simulink model "c01_MainAdc"  (R2024a)
settings: Solver=FixedStepDiscrete  StartTime=0.0  StopTime=1  FixedStep=mSim.dTime  MaxStep=Define.sModelSampleTime  RelTol=7.1420e-05
undefined symbols (not defined in the file): C01ISENS, C01VSENS, C01VTEST
libraries: Lib_LPF x1
settings Model: Creator=user  LastModifiedBy=admin
settings SolverCC: MaxConsecutiveZCs=10000  ZeroCrossAlgorithm=Adaptive  AlgebraicLoopSolver=TrustRegion
settings DataIOCC: SaveOutput=off  DSMLogging=off  InspectSignalLogs=on  SaveTime=off  SignalLoggingName=logsout_Validator
settings OptimizationCC: BlockReduction=off  DefaultParameterBehavior=Inlined  UseDivisionForNetSlopeComputation=UseDivisionForReciprocalsOfIntegersOnly  GainParamInheritBuiltInType=on  UseFloatMulNetSlope=on  DefaultUnderspecifiedDataType=single  InlineInvariantSignals=on  BitwiseOrLogicalOp=Logical operator  PassReuseOutputArgsAs=Individual arguments  EfficientFloat2IntCast=on  LifeSpan=Inf  OptimizeBlockOrder=speed  DifferentSizesBufferReuse=on  EfficientTunableParamExpr=on
settings DebuggingCC: SignalInfNanChecking=error  SignalRangeChecking=error  ReadBeforeWriteMsg=EnableAllAsError  WriteAfterWriteMsg=EnableAllAsError  WriteAfterReadMsg=EnableAllAsError  AlgebraicLoopMsg=error  ArtificialAlgebraicLoopMsg=error  SaveWithDisabledLinksMsg=error  SaveWithParameterizedLinksMsg=error  BlockPriorityViolationMsg=error  SolverPrmCheckMsg=error  InheritedTsInSrcMsg=error  SingleTaskRateTransMsg=error  TasksWithSamePriorityMsg=error  SigSpecEnsureSampleTimeMsg=error  CheckMatrixSingularityMsg=error  IntegerOverflowMsg=error  ParameterUnderflowMsg=error  ParameterPrecisionLossMsg=error  ParameterTunabilityLossMsg=error  UnderSpecifiedDataTypeMsg=error  UnnecessaryDatatypeConvMsg=warning  VectorMatrixConversionMsg=error  SignalLabelMismatchMsg=error  UnconnectedInputMsg=error  UnconnectedOutputMsg=error  UnconnectedLineMsg=error  SFcnCompatibilityMsg=error  UniqueDataStoreMsg=error  BusObjectLabelMismatch=error  RootOutportRequireBusObject=error  AssertControl=DisableAll  ModelReferenceIOMismatchMessage=error  UnknownTsInhSupMsg=error  ModelReferenceDataLoggingMessage=error  ModelReferenceSymbolNameMessage=none  StateNameClashWarn=warning  StrictBusMsg=ErrorOnBusTreatedAsVector  NonBusSignalsTreatedAsBus=error  SFInvalidInputDataAccessInChartInitDiag=error  SFTransitionOutsideNaturalParentDiag=error  SFUnreachableExecutionPathDiag=error  SFUndirectedBroadcastEventsDiag=error  SFTransitionActionBeforeConditionDiag=error  SFTemporalDelaySmallerThanSampleTimeDiag=error  SFSelfTransitionDiag=error  SFExecutionAtInitializationDiag=error  IntegerSaturationMsg=error  UnitsInconsistencyMsg=none  VariantConditionMismatch=error
settings HardwareCC: ProdBitPerChar=16  ProdBitPerInt=16  ProdBitPerPointer=32  ProdBitPerSizeT=32  ProdBitPerPtrDiffT=32  ProdLargestAtomicInteger=Integer  ProdLargestAtomicFloat=None  ProdWordSize=16  ProdLongLongMode=on  ProdHWDeviceType=Texas Instruments->C2000
settings ModelReferenceCC: EnableRefExpFcnMdlSchedulingChecks=on  ModelReferenceNumInstancesAllowed=Single
settings SFSimCC: SimUseLocalCustomCode=off  CompileTimeRecursionLimit=0  EnableRuntimeRecursion=off  MATLABDynamicMemAlloc=off  CustomCodeUndefinedFunction=UseInterfaceOnly
settings RTWCC: Description=Embedded Coder  SystemTargetFile=ert.tlc  GenCodeOnly=on  TemplateMakefile=ert_default_tmf  GenerateReport=on  RTWUseLocalCustomCode=off  BuildConfiguration=Faster Runs  IncludeHyperlinkInReport=on  LaunchReport=on  GenerateTraceInfo=on  GenerateTraceReport=on  GenerateTraceReportSl=on  GenerateTraceReportSf=on  GenerateWebview=on  GenerateCodeMetricsReport=on  GenerateCodeReplacementReport=on  GPUComputeCapability=3.5  DLArmComputeVersion=19.05
settings CodeAppCC: ForceParamTrailComments=on  IgnoreCustomStorageClasses=off  MATLABFcnDesc=on  MangleLength=4  CustomSymbolStrGlobalVar=GvC01$N$M  CustomSymbolStrType=StrC01$N$M  CustomSymbolStrFcn=$N$M$F  CustomSymbolStrMacro=$N$M  DefineNamingRule=UpperCase  ParamNamingRule=UpperCase  SimulinkBlockComments=off  MATLABSourceComments=on  EnableCustomComments=on  ReqsInCode=on
settings ERTTargetCC: TargetLangStandard=C99 (ISO)  UtilityFuncGeneration=Shared location  MultiwordLength=2048  IncludeMdlTerminateFcn=off  CombineSignalStateStructs=on  SuppressErrorStatus=on  SupportAbsoluteTime=off  SupportNonFinite=off  ParenthesesLevel=Maximum  CastingMode=Standards  GenerateSharedConstants=off  InlinedParameterPlacement=NonHierarchical  ERTSrcFileBannerTemplate=t_code_template.cgt  ERTHdrFileBannerTemplate=t_code_template.cgt  ERTDataSrcFileTemplate=t_code_template.cgt  ERTDataHdrFileTemplate=t_code_template.cgt  ERTCustomFileTemplate=example_file_process.tlc  ERTFilePackagingFormat=CompactWithDataFile  PreserveExpressionOrder=on  SuppressUnreachableDefaultCases=off  EnableSignedLeftShifts=off  EnableSignedRightShifts=off  IndentStyle=Allman  IndentSize=4
settings ConfigComp: CovSaveName=coveragedata  CovMetricSettings=we  CovEnableCumulative=off  CovSaveCumulativeToWorkspaceVar=on  CovSaveSingleToWorkspaceVar=on  CovOutputDir=sldv_output/$ModelName$\sldv_covoutput  PSVerificationMode=BugFinder  PSModelRefIgnoreList=[]  PSEnableModelRefIgnoreList=off  PSModelRefMinMaxVerif=CheckAndConstrain  PSAutoStubLUT=on  DVModelCoverageObjectives=MCDC  DVTestSuiteOptimization=CombinedObjectives (Nonlinear Extended)  DVRebuildModelRepresentation=Always
settings SimscapeCC: SimscapeNormalizeSystem=off

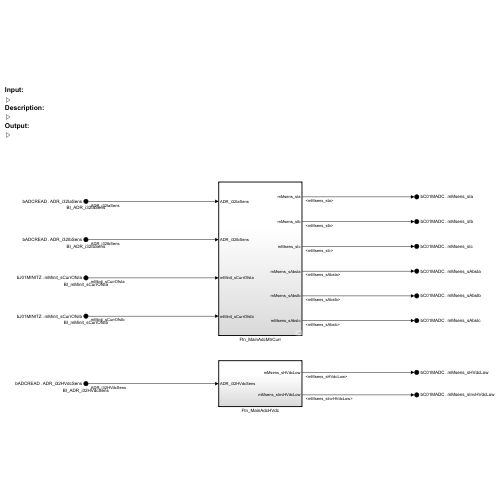
[thumbnail: Simulink's stored preview of the top-level diagram]
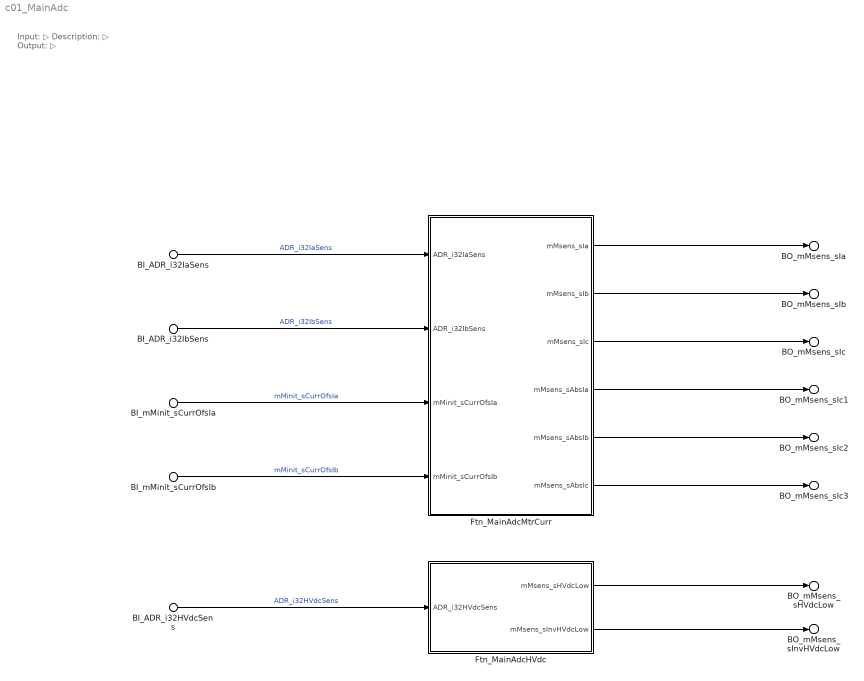
== system c01_MainAdc ==
  note: Input:
      | ▷
      | Description:
      | ▷
      | Output:
      | ▷
  BI_ADR_i32IaSens : Inport  Description=■ 설명: A상 전류 센서 ADCV  PortName=bADCREAD  Element=ADR_i32IaSens
  BI_ADR_i32IbSens : Inport  Description=■ 설명: B상 전류 센서 ADCV  PortName=bADCREAD  Element=ADR_i32IbSens
  BI_ADR_i32HVdcSens : Inport  Description=■ 설명: DC Link 전압 센서 ADCV  PortName=bADCREAD  Element=ADR_i32HVdcSens
  BI_mMinit_sCurrOfsIa : Inport  Description=■ 설명: A상 전류 센서 오프셋  Port=2  PortName=bJ01MINITZ  Element=mMinit_sCurrOfsIa
  BI_mMinit_sCurrOfsIb : Inport  Description=■ 설명: B상 전류 센서 오프셋  Port=2  PortName=bJ01MINITZ  Element=mMinit_sCurrOfsIb
  Ftn_MainAdcHVdc : Subsystem  TreatAsAtomicUnit=on
      settings: RTWSystemCode=Nonreusable function
  Ftn_MainAdcMtrCurr : Subsystem  TreatAsAtomicUnit=on
      settings: RTWSystemCode=Nonreusable function
  BO_mMsens_sIa : Outport  Description=■ 설명: A상 전류  PortName=bC01MADC  Element=mMsens_sIa
  BO_mMsens_sIb : Outport  Description=■ 설명: B상 전류  PortName=bC01MADC  Element=mMsens_sIb
  BO_mMsens_sIc : Outport  Description=■ 설명: C상 전류  PortName=bC01MADC  Element=mMsens_sIc
  BO_mMsens_sIc1 : Outport  Description=■ 설명: A상 전류 절대값  PortName=bC01MADC  Element=mMsens_sAbsIa
  BO_mMsens_sIc2 : Outport  Description=■ 설명: B상 전류 절대값  PortName=bC01MADC  Element=mMsens_sAbsIb
  BO_mMsens_sIc3 : Outport  Description=■ 설명: C상 전류 절대값  PortName=bC01MADC  Element=mMsens_sAbsIc
  BO_mMsens_sHVdcLow : Outport  Description=■ 설명: DC Link 전압  PortName=bC01MADC  Element=mMsens_sHVdcLow
  BO_mMsens_sInvHVdcLow : Outport  Description=■ 설명: DC Link 전압 역수  PortName=bC01MADC  Element=mMsens_sInvHVdcLow
  wires:
  Ftn_MainAdcMtrCurr/1(mMsens_sIa) -> BO_mMsens_sIa/1
  Ftn_MainAdcMtrCurr/3(mMsens_sIc) -> BO_mMsens_sIc/1
  Ftn_MainAdcMtrCurr/2(mMsens_sIb) -> BO_mMsens_sIb/1
  BI_ADR_i32IaSens/1 -> Ftn_MainAdcMtrCurr/1(ADR_i32IaSens)  "ADR_i32IaSens"
  BI_ADR_i32IbSens/1 -> Ftn_MainAdcMtrCurr/2(ADR_i32IbSens)  "ADR_i32IbSens"
  BI_mMinit_sCurrOfsIa/1 -> Ftn_MainAdcMtrCurr/3(mMinit_sCurrOfsIa)  "mMinit_sCurrOfsIa"
  BI_mMinit_sCurrOfsIb/1 -> Ftn_MainAdcMtrCurr/4(mMinit_sCurrOfsIb)  "mMinit_sCurrOfsIb"
  BI_ADR_i32HVdcSens/1 -> Ftn_MainAdcHVdc/1(ADR_i32HVdcSens)  "ADR_i32HVdcSens"
  Ftn_MainAdcHVdc/2(mMsens_sInvHVdcLow) -> BO_mMsens_sInvHVdcLow/1
  Ftn_MainAdcHVdc/1(mMsens_sHVdcLow) -> BO_mMsens_sHVdcLow/1
  Ftn_MainAdcMtrCurr/4(mMsens_sAbsIa) -> BO_mMsens_sIc1/1
  Ftn_MainAdcMtrCurr/5(mMsens_sAbsIb) -> BO_mMsens_sIc2/1
  Ftn_MainAdcMtrCurr/6(mMsens_sAbsIc) -> BO_mMsens_sIc3/1

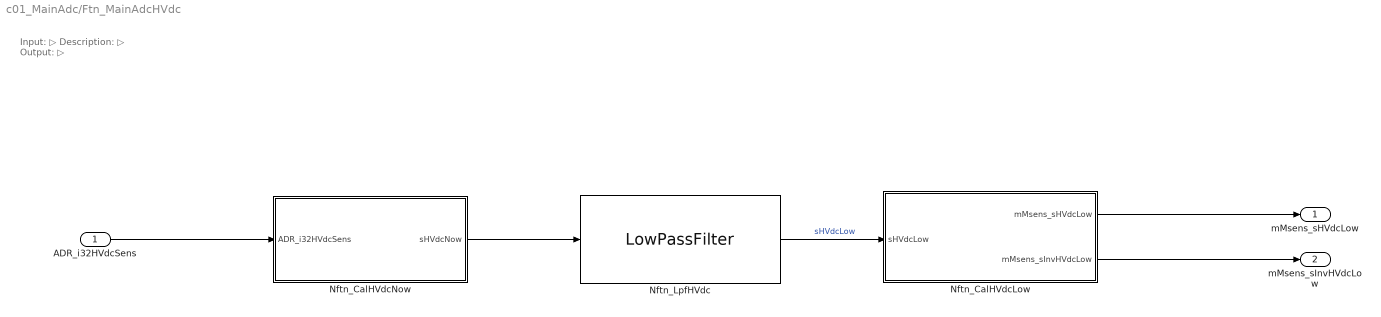
== system c01_MainAdc/Ftn_MainAdcHVdc ==
  note: Input:
      | ▷
      | Description:
      | ▷
      | Output:
      | ▷
  ADR_i32HVdcSens : Inport  Description=■ HVdc AADC 변환 값
      settings: AttributesFormatString=%<Description>
  Nftn_CalHVdcLow : Subsystem
  Nftn_CalHVdcNow : Subsystem
  Nftn_LpfHVdc : Lib_LPF/LowPassFilter  La=C01HVSWF.sHVdcLa  Lb=C01HVSWF.sHVdcLb  Init_Value=C01HVSWF.sVdcInit
  mMsens_sHVdcLow : Outport
  mMsens_sInvHVdcLow : Outport  Port=2
  wires:
  Nftn_CalHVdcNow/1(sHVdcNow) -> Nftn_LpfHVdc/1
  ADR_i32HVdcSens/1 -> Nftn_CalHVdcNow/1(ADR_i32HVdcSens)
  Nftn_CalHVdcLow/2(mMsens_sInvHVdcLow) -> mMsens_sInvHVdcLow/1
  Nftn_CalHVdcLow/1(mMsens_sHVdcLow) -> mMsens_sHVdcLow/1
  Nftn_LpfHVdc/1 -> Nftn_CalHVdcLow/1(sHVdcLow)  "sHVdcLow"

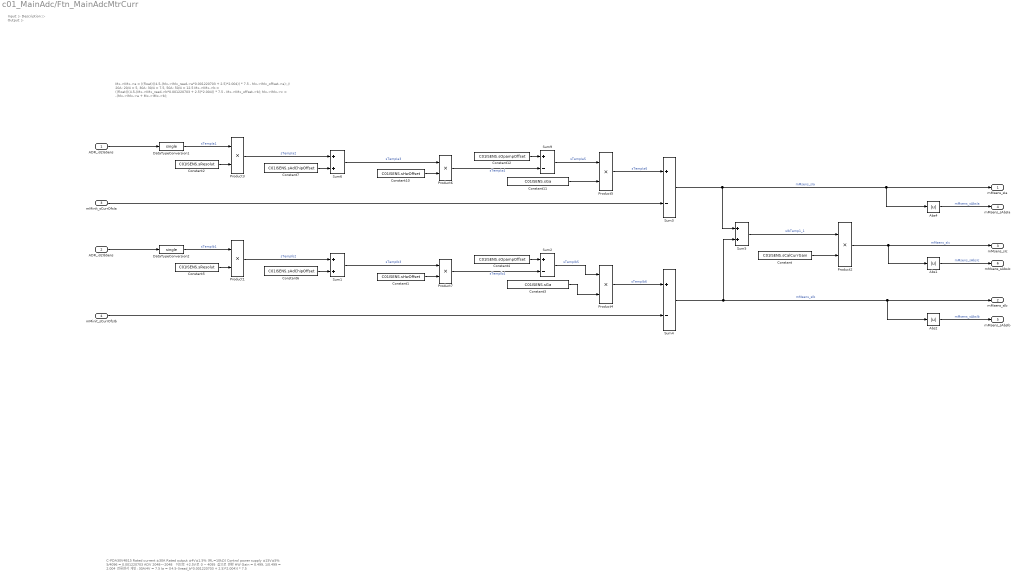
== system c01_MainAdc/Ftn_MainAdcMtrCurr ==
  note: Mx->IMx->a = ((float)((4.5-(Mx->IMx_read->a*0.001220703 + 2.5)*2.004)) * 7.5 - Mx->IMx_offset->a); // 20A: 20/4 = 5, 30A: 30/4 = 7.5, 50A: 50/4 = 12.5
      | Mx->IMx->b = ((float)((4.5-(Mx->IMx_read->b*0.001220703 + 2.5)*2.004)) * 7.5 - Mx->IMx_offset->b);
      | Mx->IMx->c = -(Mx->IMx->a + Mx->IMx->b);
  note: C-PDA30V4B15
      | Rated current ±30A
      | Rated output ±4V±1.5% (RL=10kΩ)
      | Control power supply ±15V±5%
      |
      | 5/4096 = 0.001220703
      | ADV 2048~-2048이므로 +2.5V로 0 ~ 4095 값으로 변환
      | HW Gain = 0.499, 1/0.499 = 2.004
      | 전류센서 게인: 30A/4V = 7.5
      |
      | Ia = ((4.5-(Iread_b*0.001220703 + 2.5)*2.004)) * 7.5
  note: Input:
      | ▷
      | Description:
      | ▷
      | Output:
      | ▷
  ADR_i32IaSens : Inport
  ADR_i32IbSens : Inport  Port=2
  mMinit_sCurrOfsIa : Inport  Port=3
  mMinit_sCurrOfsIb : Inport  Port=4
  Abs1 : Abs  SaturateOnIntegerOverflow=off  OutDataTypeStr=Inherit: Inherit via internal rule
  Abs2 : Abs  SaturateOnIntegerOverflow=off  OutDataTypeStr=Inherit: Inherit via internal rule
  Abs4 : Abs  SaturateOnIntegerOverflow=off  OutDataTypeStr=Inherit: Inherit via internal rule
  Constant : Constant  Value=C01ISENS.sCalCurrGain
  Constant1 : Constant  Value=C01ISENS.sHwOffset  OutDataTypeStr=single
  Constant10 : Constant  Value=C01ISENS.sHwOffset  OutDataTypeStr=single
  Constant11 : Constant  Tag=PGY  Value=C01ISENS.sGa  OutDataTypeStr=single
  Constant12 : Constant  Value=C01ISENS.sOpampOffset  OutDataTypeStr=single
  Constant2 : Constant  Value=C01ISENS.sResolut  OutDataTypeStr=single
  Constant3 : Constant  Tag=PGY  Value=C01ISENS.sGa  OutDataTypeStr=single
  Constant4 : Constant  Value=C01ISENS.sOpampOffset  OutDataTypeStr=single
  Constant5 : Constant  Value=C01ISENS.sResolut  OutDataTypeStr=single
  Constant6 : Constant  Value=C01ISENS.sAdChipOffset  OutDataTypeStr=single
  Constant7 : Constant  Value=C01ISENS.sAdChipOffset  OutDataTypeStr=single
  DataTypeConversion1 : DataTypeConversion  OutDataTypeStr=single  SaturateOnIntegerOverflow=off  RndMeth=Floor
  DataTypeConversion2 : DataTypeConversion  OutDataTypeStr=single  SaturateOnIntegerOverflow=off  RndMeth=Floor
  Product{1..7} (7 alike) : Product
  Sum1 : Sum
  Sum{2..4,9} (4 alike) : Sum  Inputs=+-
  Sum5 : Sum
  Sum6 : Sum
  mMsens_sIa : Outport
  mMsens_sIb : Outport  Port=2
  mMsens_sIc : Outport  Port=3
  mMsens_sAbsIa : Outport  Port=4
  mMsens_sAbsIb : Outport  Port=5
  mMsens_sAbsIc : Outport  Port=6
  wires:
  ADR_i32IbSens/1 -> DataTypeConversion2/1
  mMinit_sCurrOfsIb/1 -> Sum4/2
  Sum5/1 -> Product2/1  "sIbTemp1_1"
  Constant/1 -> Product2/2
  mMinit_sCurrOfsIa/1 -> Sum3/2
  Sum9/1 -> Product5/1  "sTempIa5"
  Constant12/1 -> Sum9/1
  Constant11/1 -> Product5/2
  Constant10/1 -> Product6/2
  Constant7/1 -> Sum6/2
  Constant2/1 -> Product3/2
  Product6/1 -> Sum9/2  "sTempIa4"
  Sum6/1 -> Product6/1  "sTempIa3"
  DataTypeConversion1/1 -> Product3/1  "sTempIa1"
  Product3/1 -> Sum6/1  "sTempIa2"
  Product5/1 -> Sum3/1  "sTempIa6"
  ADR_i32IaSens/1 -> DataTypeConversion1/1
  Product4/1 -> Sum4/1  "sTempIb6"
  Constant1/1 -> Product7/2
  Product1/1 -> Sum1/1  "sTempIb2"
  DataTypeConversion2/1 -> Product1/1  "sTempIb1"
  Sum1/1 -> Product7/1  "sTempIb3"
  Sum2/1 -> Product4/1  "sTempIb5"
  Constant6/1 -> Sum1/2
  Constant3/1 -> Product4/2
  Constant4/1 -> Sum2/1
  Constant5/1 -> Product1/2
  Product7/1 -> Sum2/2  "sTempIb4"
  Abs2/1 -> mMsens_sAbsIb/1  "mMsens_sAbsIb"
  Sum3/1 -> Sum5/1, Abs4/1, mMsens_sIa/1  "mMsens_sIa"
  Sum4/1 -> Abs2/1, mMsens_sIb/1, Sum5/2  "mMsens_sIb"
  Abs1/1 -> mMsens_sAbsIc/1  "mMsens_sAbsIc"
  Abs4/1 -> mMsens_sAbsIa/1  "mMsens_sAbsIa"
  Product2/1 -> Abs1/1, mMsens_sIc/1  "mMsens_sIc"

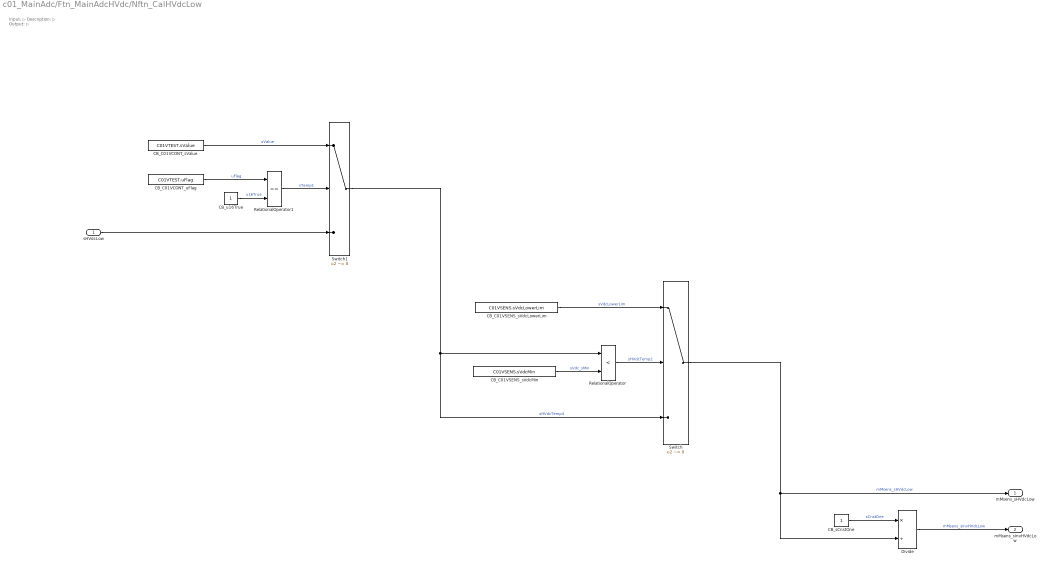
== system c01_MainAdc/Ftn_MainAdcHVdc/Nftn_CalHVdcLow ==
  note: Input:
      | ▷
      | Description:
      | ▷
      | Output:
      | ▷
  sHVdcLow : Inport
  CB_C01VCONT_sValue : Constant  Value=C01VTEST.sValue
  CB_C01VCONT_uFlag : Constant  Value=C01VTEST.uFlag
  CB_C01VSENS_sVdcLowerLim : Constant  Value=C01VSENS.sVdcLowerLim
  CB_C01VSENS_sVdcMin : Constant  Value=C01VSENS.sVdcMin
  CB_sCnstOne : Constant  OutDataTypeStr=single
  CB_u16True : Constant  OutDataTypeStr=uint16
  Divide : Product  Inputs=*/
  RelationalOperator : RelationalOperator  Operator=<  RndMeth=Simplest  InputSameDT=off
  RelationalOperator1 : RelationalOperator  Operator===  RndMeth=Simplest  InputSameDT=off
  Switch : Switch  Criteria=u2 ~= 0  SaturateOnIntegerOverflow=off  InputSameDT=off
  Switch1 : Switch  Criteria=u2 ~= 0  SaturateOnIntegerOverflow=off  InputSameDT=off
  mMsens_sHVdcLow : Outport
  mMsens_sInvHVdcLow : Outport  Port=2
  wires:
  Divide/1 -> mMsens_sInvHVdcLow/1  "mMsens_sInvHVdcLow"
  CB_C01VSENS_sVdcLowerLim/1 -> Switch/1  "sVdcLowerLim"
  Switch1/1 -> Switch/3, RelationalOperator/1  "sHVdcTemp4"
  CB_sCnstOne/1 -> Divide/1  "sCnstOne"
  CB_C01VSENS_sVdcMin/1 -> RelationalOperator/2  "sVdc_sMin"
  Switch/1 -> Divide/2, mMsens_sHVdcLow/1  "mMsens_sHVdcLow"
  RelationalOperator/1 -> Switch/2  "sHVdcTemp2"
  RelationalOperator1/1 -> Switch1/2  "sTemp1"
  CB_C01VCONT_sValue/1 -> Switch1/1  "sValue"
  sHVdcLow/1 -> Switch1/3
  CB_u16True/1 -> RelationalOperator1/2  "u16True"
  CB_C01VCONT_uFlag/1 -> RelationalOperator1/1  "uFlag"

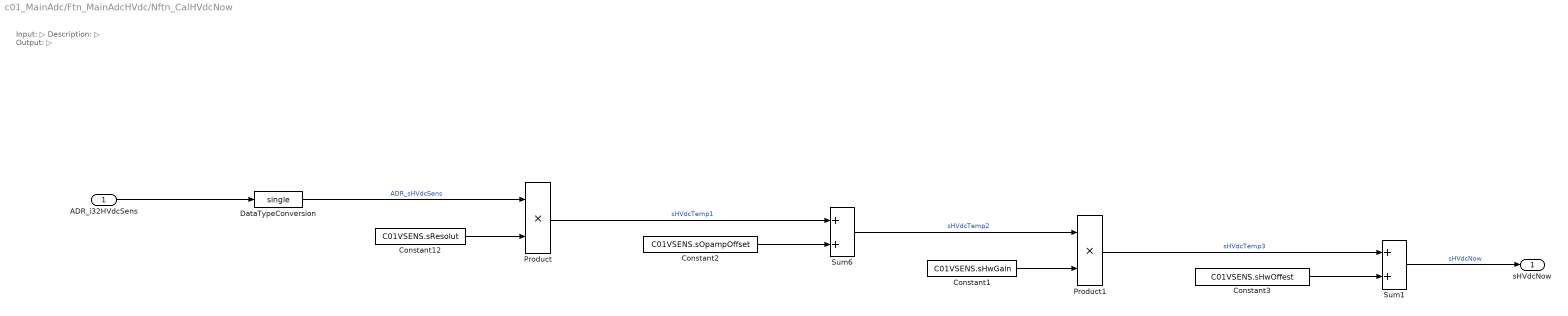
== system c01_MainAdc/Ftn_MainAdcHVdc/Nftn_CalHVdcNow ==
  note: Input:
      | ▷
      | Description:
      | ▷
      | Output:
      | ▷
  ADR_i32HVdcSens : Inport
  Constant1 : Constant  Value=C01VSENS.sHwGain  OutDataTypeStr=single
  Constant12 : Constant  Value=C01VSENS.sResolut  OutDataTypeStr=single
  Constant2 : Constant  Value=C01VSENS.sOpampOffset  OutDataTypeStr=single
  Constant3 : Constant  Value=C01VSENS.sHwOffest  OutDataTypeStr=single
  DataTypeConversion : DataTypeConversion  OutDataTypeStr=single  SaturateOnIntegerOverflow=off  RndMeth=Floor
  Product : Product
  Product1 : Product
  Sum1 : Sum
  Sum6 : Sum
  sHVdcNow : Outport
  wires:
  Sum6/1 -> Product1/1  "sHVdcTemp2"
  ADR_i32HVdcSens/1 -> DataTypeConversion/1
  Constant2/1 -> Sum6/2
  Constant1/1 -> Product1/2
  Product/1 -> Sum6/1  "sHVdcTemp1"
  Constant3/1 -> Sum1/2
  Product1/1 -> Sum1/1  "sHVdcTemp3"
  Constant12/1 -> Product/2
  DataTypeConversion/1 -> Product/1  "ADR_sHVdcSens"
  Sum1/1 -> sHVdcNow/1  "sHVdcNow"
